simulink model "PubIfDecisionTOS_MDL"  (R2020b)
settings: configuration reference "DspaceConfig" (kept outside this file)
PostLoadFcn:
  | if any(exist('dsrtsu_mdlpostloadfcn', 'file') ~= 0), dsrtsu_mdlpostloadfcn('Execute', bdroot); end
InitFcn:
  | , if any(exist('dsmpb_private', 'file') ~= 0), dsmpb_private('dsmpb_mdlclblib', 'Init', bdroot); end,
undefined symbols (not defined in the file or in its folder): C_TOS_ACCEgoRAxletoFbumplength_m, C_TOS_ACCTargetFront_Flag, C_TOS_AEBJAPedObjDxThre_Val, C_TOS_AEBJAPedObjDyThre_Val, C_TOS_AEBJATargetSize_Val, C_TOS_AEBJAVehObjDxThre_Val, C_TOS_AEBJAVehObjDyThre_Val, C_TOS_AEBJuncPedTargetSize_Val, C_TOS_AEBLatObjDxThre_Val, C_TOS_AEBLatPedDyThre_Val, C_TOS_AEBLatTargetSize_Val, C_TOS_AEBLongTargetInEgoFront_Flag, C_TOS_axAbsGround_Parameter, C_TOS_CameraConfirmedFlag, C_TOS_CNsubjWidth, C_TOS_CurrentLaneCoreMinWidth_Val, C_TOS_CutInProb_Val_Zero, C_TOS_CutOutProb_Val_Zero, C_TOS_D2R_Val, C_TOS_DefaultValueObjectToCenterLine_dy, C_TOS_EgoCarWidth_Val, C_TOS_EgoDxRefPoint_m, C_TOS_EgoRAxletoFbumplength_m, C_TOS_HalfWidthVehicle_Con, C_TOS_HWA_CurrentLaneFlag, C_TOS_HWA_LeftLaneFlag, C_TOS_HWA_MovingDir_Vaild, C_TOS_HWA_MovState_Vaild, C_TOS_HWA_RightLaneFlag, C_TOS_LaneLineCourseErrorFront, C_TOS_LaneLineCourseErrorRear, C_TOS_MotorbikeDefaultWidth_m, C_TOS_NumberOfEffectiveTargets, C_TOS_Obj_Age_Val, C_TOS_Objdx_Constraint_Val, C_TOS_ObjectDefaultWidth_m, C_TOS_ObjInCurrentLane_Val, C_TOS_ObjInCurrentLaneValid, C_TOS_ObjInLeftLaneValid, C_TOS_ObjInRightLaneValid, C_TOS_ObjNotInCurrentLane_Val, C_TOS_ObjNotREElementType, C_TOS_ObjPredictDis_dy_ConstantVal_Zeros, C_TOS_ObjToCenterLine_ConstantVal_Zeros, C_TOS_OFMObjIDInvilad_Val, C_TOS_PIL_LatDisCons_Val_zero, C_TOS_PIL_ObjectCutInFlag_b, C_TOS_PIL_ObjectCutOutFlag_b, C_TOS_PIL_ObjLaneProb_al_Val, C_TOS_PP_ObjFusType_FC_Confirm_b, C_TOS_PP_ObjFusType_FC_FR_Confirm_b, C_TOS_PP_ObjFusType_FR_Confirm_b, C_TOS_RE_80BoolDefault_Val, C_TOS_RE_80Single181Default_Val, C_TOS_RE_80Single255Default_Val, C_TOS_RE_80Uint8Default_Val, C_TOS_RE_D2R, C_TOS_RE_D_180_Val, C_TOS_RE_InvalidObjectID_Val, C_TOS_RE_InvalidTargetChainDir_Val ... (+142)
libraries: simulink x1650, TOS_LIB x361, canfdmsglib x14
(part 15 of 69)

== system PubIfDecisionTOS_MDL/TOS_20201112/TOS_2012080320/PIL_1029/BoundaryCalculat/ObjectToCenterLine_dyc/SameLane/PIL_ObjectToCenterLine_dy_Filt ==
  note: fun: 目标到本车道中心线距离滤波
  TOS_OFMObjValid_Flag : Inport
  Object_ID : Inport  Port=2  OutDataTypeStr=uint8
  Object_Age : Inport  Port=3
  ObjectToCenterLine_dy : Inport  Port=4
  PIL_ObjectToCenterLine_dy : Subsystem
  Unit Delay : UnitDelay  InitialCondition=zeros(80,1)  SampleTime=-1  HasFrameUpgradeWarning=on
      settings: AttributesFormatString=initVal = zeros(80,1)
  Unit Delay1 : UnitDelay  InitialCondition=ones(80,1)*255  SampleTime=-1  HasFrameUpgradeWarning=on
      settings: AttributesFormatString=initVal = ones(80,1)*255
  PIL_ObjectToCenterLine_dy_Filt : Outport  OutDataTypeStr=single
  wires:
  TOS_OFMObjValid_Flag/1 -> PIL_ObjectToCenterLine_dy/4(TOS_OFMObjValid_Flag)
  Object_Age/1 -> PIL_ObjectToCenterLine_dy/6(Object_Age)
  ObjectToCenterLine_dy/1 -> PIL_ObjectToCenterLine_dy/3(ObjectToCenterLine_dy)
  PIL_ObjectToCenterLine_dy/2(ObjectToCenterLine_dy_Filt) -> PIL_ObjectToCenterLine_dy_Filt/1, Unit Delay1/1
  Unit Delay1/1 -> PIL_ObjectToCenterLine_dy/2(ObjectToCenterLine_dy_Filt_K1)
  Object_ID/1 -> PIL_ObjectToCenterLine_dy/5(Object_ID)
  PIL_ObjectToCenterLine_dy/1(Obj_ID) -> Unit Delay/1
  Unit Delay/1 -> PIL_ObjectToCenterLine_dy/1(ObjectID_Filt_K1)

== system PubIfDecisionTOS_MDL/TOS_20201112/TOS_2012080320/PIL_1029/BoundaryCalculat/ObjectToCenterLine_dyc/SameLane/SameCenterLine_dyc ==
  TOS_OFMObjValid_Flag : Inport  Partition=on  PartitionDimension=1  PartitionWidth=1  PartitionOffset=0
  Object_DY : Inport  Port=2  Partition=on  PartitionDimension=1  PartitionWidth=1  PartitionOffset=0
  Object_DX : Inport  Port=3  Partition=on  PartitionDimension=1  PartitionWidth=1  PartitionOffset=0
  line01_C0 : Inport  Port=4
  line01_C1 : Inport  Port=5
  line01_C2 : Inport  Port=6
  line01_C3 : Inport  Port=7
  line01_dDisStart : Inport  Port=8
  line01_dDisEnd : Inport  Port=9
  line02_C0 : Inport  Port=10
  line02_C1 : Inport  Port=11
  line02_C2 : Inport  Port=12
  line02_C3 : Inport  Port=13
  line02_dDisStart : Inport  Port=14
  line02_dDisEnd : Inport  Port=15
  line03_C0 : Inport  Port=16
  line03_C1 : Inport  Port=17
  line03_C2 : Inport  Port=18
  line03_C3 : Inport  Port=19
  line03_dDisStart : Inport  Port=20
  line03_dDisEnd : Inport  Port=21
  line04_C0 : Inport  Port=22
  line04_C1 : Inport  Port=23
  line04_C2 : Inport  Port=24
  line04_C3 : Inport  Port=25
  line04_dDisStart : Inport  Port=26
  line04_dDisEnd : Inport  Port=27
  line05_C0 : Inport  Port=28
  line05_C1 : Inport  Port=29
  line05_C2 : Inport  Port=30
  line05_C3 : Inport  Port=31
  line05_dDisStart : Inport  Port=32
  line05_dDisEnd : Inport  Port=33
  line06_C0 : Inport  Port=34
  line06_C1 : Inport  Port=35
  line06_C2 : Inport  Port=36
  line06_C3 : Inport  Port=37
  line06_dDisStart : Inport  Port=38
  line06_dDisEnd : Inport  Port=39
  Compare To Constant : simulink/Logic and Bit Operations/Compare To Constant  relop===  const=C_TOS_OFMObjIDInvilad_Val  OutDataTypeStr=boolean
      settings: AttributesFormatString=C_TOS_OFMObjIDInvilad_Val = 0
  For Each : ForEach  DisableCoverage=on
  If : If  IfExpression=u1 ~= 0
  Merge : Merge
  ObjToCenterLine_dyc_CurrentLane : Subsystem
  ObjToCenterLine_dyc_CurrentLaneDefault : Subsystem  TreatAsAtomicUnit=on
  SameCenterLine_dyc : Outport  ConcatenationDimension=1
  wires:
  ObjToCenterLine_dyc_CurrentLaneDefault/1(ObjectToCenterLine_dyc_CurrentLane) -> Merge/1
  Merge/1 -> SameCenterLine_dyc/1
  TOS_OFMObjValid_Flag/1 -> Compare To Constant/1
  If/2 -> ObjToCenterLine_dyc_CurrentLane/Action
  Compare To Constant/1 -> If/1
  If/1 -> ObjToCenterLine_dyc_CurrentLaneDefault/Action
  ObjToCenterLine_dyc_CurrentLane/1(ObjectToCenterLine_dyc_CurrentLane) -> Merge/2
  line06_dDisEnd/1 -> ObjToCenterLine_dyc_CurrentLane/38(line06_dDisEnd)
  line06_dDisStart/1 -> ObjToCenterLine_dyc_CurrentLane/37(line06_dDisStart)
  line06_C3/1 -> ObjToCenterLine_dyc_CurrentLane/36(line06_C3)
  line06_C2/1 -> ObjToCenterLine_dyc_CurrentLane/35(line06_C2)
  line06_C1/1 -> ObjToCenterLine_dyc_CurrentLane/34(line06_C1)
  line06_C0/1 -> ObjToCenterLine_dyc_CurrentLane/33(line06_C0)
  line05_dDisEnd/1 -> ObjToCenterLine_dyc_CurrentLane/32(line05_dDisEnd)
  line05_dDisStart/1 -> ObjToCenterLine_dyc_CurrentLane/31(line05_dDisStart)
  line05_C3/1 -> ObjToCenterLine_dyc_CurrentLane/30(line05_C3)
  line05_C2/1 -> ObjToCenterLine_dyc_CurrentLane/29(line05_C2)
  line05_C1/1 -> ObjToCenterLine_dyc_CurrentLane/28(line05_C1)
  line05_C0/1 -> ObjToCenterLine_dyc_CurrentLane/27(line05_C0)
  line04_dDisEnd/1 -> ObjToCenterLine_dyc_CurrentLane/26(line04_dDisEnd)
  line04_dDisStart/1 -> ObjToCenterLine_dyc_CurrentLane/25(line04_dDisStart)
  line04_C3/1 -> ObjToCenterLine_dyc_CurrentLane/24(line04_C3)
  line04_C2/1 -> ObjToCenterLine_dyc_CurrentLane/23(line04_C2)
  line04_C1/1 -> ObjToCenterLine_dyc_CurrentLane/22(line04_C1)
  line04_C0/1 -> ObjToCenterLine_dyc_CurrentLane/21(line04_C0)
  line03_dDisEnd/1 -> ObjToCenterLine_dyc_CurrentLane/20(line03_dDisEnd)
  line03_dDisStart/1 -> ObjToCenterLine_dyc_CurrentLane/19(line03_dDisStart)
  line03_C3/1 -> ObjToCenterLine_dyc_CurrentLane/18(line03_C3)
  line03_C2/1 -> ObjToCenterLine_dyc_CurrentLane/17(line03_C2)
  line03_C1/1 -> ObjToCenterLine_dyc_CurrentLane/16(line03_C1)
  line03_C0/1 -> ObjToCenterLine_dyc_CurrentLane/15(line03_C0)
  line02_dDisEnd/1 -> ObjToCenterLine_dyc_CurrentLane/14(line02_dDisEnd)
  line02_dDisStart/1 -> ObjToCenterLine_dyc_CurrentLane/13(line02_dDisStart)
  line02_C3/1 -> ObjToCenterLine_dyc_CurrentLane/12(line02_C3)
  line02_C2/1 -> ObjToCenterLine_dyc_CurrentLane/11(line02_C2)
  line02_C1/1 -> ObjToCenterLine_dyc_CurrentLane/10(line02_C1)
  line02_C0/1 -> ObjToCenterLine_dyc_CurrentLane/9(line02_C0)
  line01_dDisEnd/1 -> ObjToCenterLine_dyc_CurrentLane/8(line01_dDisEnd)
  line01_dDisStart/1 -> ObjToCenterLine_dyc_CurrentLane/7(line01_dDisStart)
  line01_C3/1 -> ObjToCenterLine_dyc_CurrentLane/6(line01_C3)
  line01_C2/1 -> ObjToCenterLine_dyc_CurrentLane/5(line01_C2)
  line01_C1/1 -> ObjToCenterLine_dyc_CurrentLane/4(line01_C1)
  line01_C0/1 -> ObjToCenterLine_dyc_CurrentLane/3(line01_C0)
  Object_DX/1 -> ObjToCenterLine_dyc_CurrentLane/2(Object_DX)
  Object_DY/1 -> ObjToCenterLine_dyc_CurrentLane/1(Object_DY)

== system PubIfDecisionTOS_MDL/TOS_20201112/TOS_2012080320/PIL_1029/ObjCutInOut_Prob/ObjectCutIn/CutInProb_Calculate/CutInProb_CalculateDefault ==
  Action Port : ActionPort  ActionPortLabel=if(u1 ~= 0)
  Constant1 : Constant  Value=0  OutDataTypeStr=single
  Constant2 : Constant  Value=0  OutDataTypeStr=single
  Constant3 : Constant  Value=255  OutDataTypeStr=single
  Constant4 : Constant  Value=0  OutDataTypeStr=boolean
  Constant5 : Constant  Value=255  OutDataTypeStr=single
  PIL_CutInPredictTime_ObserVale : Outport  OutDataTypeStr=single
  PIL_CutInPredictTime_dxConstraint_ObserVale : Outport  Port=2  OutDataTypeStr=single
  PIL_CutInPredictDis_dy_ObjWidthConstraint_ObserVale : Outport  Port=3
  PIL_ObjectCutinMindFlg_ObserVale : Outport  Port=4  OutDataTypeStr=boolean
  CutInProb_Calculate : Outport  Port=5
  wires:
  Constant2/1 -> PIL_CutInPredictTime_ObserVale/1
  Constant1/1 -> PIL_CutInPredictTime_dxConstraint_ObserVale/1
  Constant3/1 -> PIL_CutInPredictDis_dy_ObjWidthConstraint_ObserVale/1
  Constant4/1 -> PIL_ObjectCutinMindFlg_ObserVale/1
  Constant5/1 -> CutInProb_Calculate/1

== system PubIfDecisionTOS_MDL/TOS_20201112/TOS_2012080320/PIL_1029/ObjCutInOut_Prob/ObjectCutIn/CutInProb_Calculate/CutInProb_Calculate_ ==
  Object_Width : Inport  OutDataTypeStr=single
  Object_DX : Inport  Port=2  OutDataTypeStr=single
  Object_DY : Inport  Port=3  OutDataTypeStr=single
  Object_Age : Inport  Port=4  OutDataTypeStr=uint16
  Object_Type : Inport  Port=5
  PP_ObjectToCenterLine_dy : Inport  Port=6  OutDataTypeStr=single
  PP_ObjectToCenterLine_vyc : Inport  Port=7  OutDataTypeStr=single
  PIL_ObjectToCenterLine_dy_Filt : Inport  Port=8  OutDataTypeStr=single
  PP_CurrentLaneWidth : Inport  Port=9
  Action Port : ActionPort  ActionPortLabel=else
  Bus Creator : BusCreator  Inputs=9
  Bus Selector : BusSelector  OutputSignals=PIL_ObjectToCenterLine_dy_Filt,PP_ObjectToCenterLine_dy,Object_Type,Object_DX,PP_ObjectToCenterLine_vyc
  Bus Selector1 : BusSelector  OutputSignals=PP_ObjectToCenterLine_dy,Object_Width,Object_Type
  Bus Selector3 : BusSelector  OutputSignals=PP_ObjectToCenterLine_vyc,PP_ObjectToCenterLine_dy,PP_ObjectToCenterLine_dy,Object_Age,Object_Width
  CutInPredictDis_dy : Subsystem
  CutInProb : Subsystem
  CutInProb_ScopeConstraint : Subsystem
  CutInProb_ScopeConstraint1 : Subsystem  Commented=on
  PIL_CutInPredictTime_ObserVale : Outport  OutDataTypeStr=single
  PIL_CutInPredictTime_dxConstraint_ObserVale : Outport  Port=2  OutDataTypeStr=single
  PIL_CutInPredictDis_dy_ObjWidthConstraint_ObserVale : Outport  Port=3
  PIL_ObjectCutinMindFlg_ObserVale : Outport  Port=4  OutDataTypeStr=boolean
  CutInProb_Calculate : Outport  Port=5
  wires:
  Bus Selector1/3 -> CutInProb/4(ObjectType)  "<Object_Type>"
  CutInProb/2(CutInProb) -> CutInProb_ScopeConstraint/1(CutInProb)  "CutInProb"
  CutInProb/1(PIL_CutInPredictDis_dy_ObjWidthConstraint_ObserVale) -> PIL_CutInPredictDis_dy_ObjWidthConstraint_ObserVale/1
  PP_ObjectToCenterLine_vyc/1 -> Bus Creator/7  "PP_ObjectToCenterLine_vyc"
  Object_Age/1 -> Bus Creator/4  "Object_Age"
  CutInPredictDis_dy/3(CutInPredictDis_dy) -> CutInProb/1(CutInPredictDis_dy)  "CutInPredictDis_dy"
  Bus Selector1/2 -> CutInProb/3(Object_Width)  "<Object_Width>"
  CutInPredictDis_dy/2(PIL_CutInPredictTime_Constraint_ObserVale) -> PIL_CutInPredictTime_dxConstraint_ObserVale/1
  Bus Selector/1 -> CutInPredictDis_dy/1(ObjectToCenterLine_dy_Filt)  "<PIL_ObjectToCenterLine_dy_Filt>"
  Object_DY/1 -> Bus Creator/3  "Object_DY"
  Bus Selector/2 -> CutInPredictDis_dy/2(ObjectToCenterLine_dy)  "<PP_ObjectToCenterLine_dy>"
  Bus Selector1/1 -> CutInProb/2(ObjectToCenterLine_dy)  "<PP_ObjectToCenterLine_dy>"
  Bus Selector3/5 -> CutInProb_ScopeConstraint/6(Object_Width)  "<Object_Width>"
  [CutInProb_Calculate] -> Bus Selector3/1
  Bus Selector3/2 -> CutInProb_ScopeConstraint/3(ObjectToCenterLine_dy)  "<PP_ObjectToCenterLine_dy>"
  Bus Selector3/3 -> CutInProb_ScopeConstraint/4(PP_ObjectToCenterLine_dy)  "<PP_ObjectToCenterLine_dy>"
  Bus Selector3/4 -> CutInProb_ScopeConstraint/5(Object_Age)  "<Object_Age>"
  Bus Selector/4 -> CutInPredictDis_dy/4(Object_DX)  "<Object_DX>"
  Bus Selector/3 -> CutInPredictDis_dy/3(ObjectType)  "<Object_Type>"
  CutInProb_ScopeConstraint/1(PIL_ObjectCutinMindFlg_ObserVale) -> PIL_ObjectCutinMindFlg_ObserVale/1
  Object_Width/1 -> Bus Creator/1  "Object_Width"
  [CutInProb_Calculate] -> Bus Selector1/1
  CutInPredictDis_dy/1(PIL_CutInPredictTime_ObserVale) -> PIL_CutInPredictTime_ObserVale/1
  Object_Type/1 -> Bus Creator/5  "Object_Type"
  Bus Selector3/1 -> CutInProb_ScopeConstraint/2(PP_ObjectToCenterLine_vyc)  "<PP_ObjectToCenterLine_vyc>"
  Bus Creator/1 -> [CutInProb_Calculate], Bus Selector/1
  PP_ObjectToCenterLine_dy/1 -> Bus Creator/6  "PP_ObjectToCenterLine_dy"
  Object_DX/1 -> Bus Creator/2  "Object_DX"
  PIL_ObjectToCenterLine_dy_Filt/1 -> Bus Creator/8  "PIL_ObjectToCenterLine_dy_Filt"
  Bus Selector/5 -> CutInPredictDis_dy/5(PP_ObjectToCenterLine_vyc)  "<PP_ObjectToCenterLine_vyc>"
  CutInProb_ScopeConstraint/2(CutInProb_ScopeConstraint) -> CutInProb_Calculate/1
  PP_CurrentLaneWidth/1 -> Bus Creator/9  "PP_CurrentLaneWidth"

== system PubIfDecisionTOS_MDL/TOS_20201112/TOS_2012080320/PIL_1029/ObjCutInOut_Prob/ObjectCutIn/CutInProb_Pluse/CutInProb_Pluse ==
  note: 滤波处理
  CutInProb_Pluse_K1 : Inport  OutDataTypeStr=single
  CutInProb_ScopeConstraint : Inport  Port=2  OutDataTypeStr=single
  Object_Dx : Inport  Port=3  OutDataTypeStr=single
  Action Port : ActionPort  ActionPortLabel=if(u1 == 1)
  1-D Lookup Table : Lookup_n-D  NumberOfTableDimensions=1  BreakpointsForDimension1=[0,10,30,100]  Table=[0.25,0.25,0.4,0.4]  InternalRulePriority=Speed  RndMeth=Simplest  InputSameDT=on
  Abs : Abs  OutDataTypeStr=single
  Abs1 : Abs  OutDataTypeStr=single
  Add : Sum  Inputs=-+  AccumDataTypeStr=single
  Add1 : Sum  AccumDataTypeStr=single
  Add2 : Sum  Inputs=+-  AccumDataTypeStr=single
  Delay : Delay
  K_CutInPluseRate_Val : Constant  Value=P_TOS_CutInPluseUpperRate_Val
      settings: AttributesFormatString=P_TOS_CutInPluseUpperRate_Val = 0.7
  K_CutInPluseRate_Val1 : Constant  Value=P_TOS_CutInPluseDecreaseRate_Val
      settings: AttributesFormatString=P_TOS_CutInPluseDecreaseRate_Val = 0.2
  Logical Operator : Logic  Inputs=3  AllPortsSameDT=off  OutDataTypeStr=boolean
  Product : Product
  Product1 : Product
  Relational Operator2 : RelationalOperator  Operator=>  OutDataTypeStr=boolean  RndMeth=Nearest
  Switch : Switch  Criteria=u2 > Threshold  OutDataTypeStr=single
  Unit Delay : UnitDelay  SampleTime=-1  HasFrameUpgradeWarning=on
  PIL_CutInProb_Pluse : Outport  OutDataTypeStr=single
  PIL_ObjectCutInFlag : Outport  Port=2
  wires:
  Logical Operator/1 -> PIL_ObjectCutInFlag/1
  Delay/1 -> Logical Operator/3
  Unit Delay/1 -> Logical Operator/2
  Add/1 -> Abs1/1, Switch/2, Abs/1
  CutInProb_Pluse_K1/1 -> Add/1, Add2/1, Add1/1
  Switch/1 -> PIL_CutInProb_Pluse/1, Relational Operator2/1
  Add2/1 -> Switch/3
  K_CutInPluseRate_Val1/1 -> Product1/2
  Add1/1 -> Switch/1
  Abs/1 -> Product/2
  Object_Dx/1 -> 1-D Lookup Table/1
  Relational Operator2/1 -> Logical Operator/1, Delay/1, Unit Delay/1
  Product1/1 -> Add2/2
  CutInProb_ScopeConstraint/1 -> Add/2
  K_CutInPluseRate_Val/1 -> Product/1
  Abs1/1 -> Product1/1
  Product/1 -> Add1/2
  1-D Lookup Table/1 -> Relational Operator2/2  "P_TOS_ObjCutInProb_Val"

== system PubIfDecisionTOS_MDL/TOS_20201112/TOS_2012080320/PIL_1029/ObjCutInOut_Prob/ObjectCutIn/CutInProb_Pluse/CutInProb_PluseDefault ==
  Action Port : ActionPort  ActionPortLabel=else
  Constant1 : Constant  Value=0  OutDataTypeStr=boolean
  Constant2 : Constant  Value=0  OutDataTypeStr=single
  PIL_CutInProb_Pluse : Outport  OutDataTypeStr=single
  PIL_ObjectCutInFlag : Outport  Port=2
  wires:
  Constant2/1 -> PIL_CutInProb_Pluse/1
  Constant1/1 -> PIL_ObjectCutInFlag/1

== system PubIfDecisionTOS_MDL/TOS_20201112/TOS_2012080320/PIL_1029/ObjCutInOut_Prob/ObjectCutOut/CutOutProb_Calculate/CutOutProb_Calculate ==
  Object_Width : Inport
  Object_DX : Inport  Port=2
  Object_DY : Inport  Port=3
  Object_Age : Inport  Port=4
  Object_Type : Inport  Port=5
  PP_ObjectToCenterLine_dy : Inport  Port=6
  PP_ObjectToCenterLine_vyc : Inport  Port=7
  PIL_ObjectToCenterLine_dy_Filt : Inport  Port=8
  Object_VY : Inport  Port=9
  Action Port : ActionPort  ActionPortLabel=else
  Bus Creator : BusCreator  Inputs=9
  Bus Selector : BusSelector  OutputSignals=PIL_ObjectToCenterLine_dy_Filt,PP_ObjectToCenterLine_dy,Object_Type,Object_DX,PP_ObjectToCenterLine_vyc,Object_VY
  Bus Selector1 : BusSelector  OutputSignals=PIL_ObjectToCenterLine_dy_Filt,Object_Width,Object_Type
  Bus Selector3 : BusSelector  OutputSignals=PIL_ObjectToCenterLine_dy_Filt,PP_ObjectToCenterLine_vyc,PP_ObjectToCenterLine_dy,Object_Width,Object_Type
  CutOutPredictDis_dy : Subsystem
  CutOutProb : Subsystem
  CutOutProb_ScopeConstraint : Subsystem
  PIL_CutOutPredictTime_ObserVale : Outport  OutDataTypeStr=single
  PIL_CutOutPredictTime_dxConstraint_ObserVale : Outport  Port=2  OutDataTypeStr=single
  PIL_CutOutPredictDis_dy_ObjWidthConstraint_ObserVale : Outport  Port=3
  PIL_ObjectCutOutMindFlg_ObserVale : Outport  Port=4  OutDataTypeStr=boolean
  PIL_CutOutProb_ScopeConstraint : Outport  Port=5
  PIL_ObjectCutoutMindFlg1_ObserVale : Outport  Port=6  OutDataTypeStr=boolean
  PIL_ObjectCutoutMindFlg2_ObserVale : Outport  Port=7  OutDataTypeStr=boolean
  PIL_ObjectCutoutMindFlg3_ObserVale : Outport  Port=8  OutDataTypeStr=boolean
  wires:
  Bus Selector3/5 -> CutOutProb_ScopeConstraint/6(ObjectType)  "<Object_Type>"
  Bus Selector/6 -> CutOutPredictDis_dy/6(Object_VY)  "<Object_VY>"
  Object_VY/1 -> Bus Creator/9  "Object_VY"
  Bus Selector3/1 -> CutOutProb_ScopeConstraint/2(PIL_ObjectToCenterLine_dy_Filt)  "<PIL_ObjectToCenterLine_dy_Filt>"
  Bus Selector1/3 -> CutOutProb/4(ObjectType)  "<Object_Type>"
  CutOutPredictDis_dy/2(PIL_CutOutPredictTime_dxConstraint_ObserVale) -> PIL_CutOutPredictTime_dxConstraint_ObserVale/1
  PP_ObjectToCenterLine_vyc/1 -> Bus Creator/7  "PP_ObjectToCenterLine_vyc"
  PP_ObjectToCenterLine_dy/1 -> Bus Creator/6  "PP_ObjectToCenterLine_dy"
  Bus Selector3/3 -> CutOutProb_ScopeConstraint/4(PP_ObjectToCenterLine_dy)  "<PP_ObjectToCenterLine_dy>"
  Bus Selector1/1 -> CutOutProb/2(PIL_ObjectToCenterLine_dy_Filt)  "<PIL_ObjectToCenterLine_dy_Filt>"
  CutOutPredictDis_dy/3(CutOutPredictDis_dy) -> CutOutProb/1(CutOutPredictDis_dy)
  Bus Selector/2 -> CutOutPredictDis_dy/2(ObjectToCenterLine_dy)  "<PP_ObjectToCenterLine_dy>"
  Object_Age/1 -> Bus Creator/4  "Object_Age"
  PIL_ObjectToCenterLine_dy_Filt/1 -> Bus Creator/8  "PIL_ObjectToCenterLine_dy_Filt"
  Bus Selector/5 -> CutOutPredictDis_dy/5(PP_ObjectToCenterLine_vyc)  "<PP_ObjectToCenterLine_vyc>"
  Bus Selector/3 -> CutOutPredictDis_dy/3(ObjectType)  "<Object_Type>"
  Bus Selector/4 -> CutOutPredictDis_dy/4(Object_DX)  "<Object_DX>"
  [CutOutProb_Calculate] -> Bus Selector3/1
  CutOutPredictDis_dy/1(PIL_CutOutPredictTime_ObserVale) -> PIL_CutOutPredictTime_ObserVale/1
  Bus Selector1/2 -> CutOutProb/3(Object_Width)  "<Object_Width>"
  Object_Type/1 -> Bus Creator/5  "Object_Type"
  Object_Width/1 -> Bus Creator/1  "Object_Width"
  Bus Selector3/2 -> CutOutProb_ScopeConstraint/3(PP_ObjectToCenterLine_vyc)  "<PP_ObjectToCenterLine_vyc>"
  Bus Selector/1 -> CutOutPredictDis_dy/1(ObjectToCenterLine_dy_Filt)  "<PIL_ObjectToCenterLine_dy_Filt>"
  Bus Creator/1 -> [CutOutProb_Calculate], Bus Selector/1
  Object_DX/1 -> Bus Creator/2  "Object_DX"
  Bus Selector3/4 -> CutOutProb_ScopeConstraint/5(Object_Width)  "<Object_Width>"
  CutOutProb/2(CutOutProb) -> CutOutProb_ScopeConstraint/1(CutOutProb)  "CutOutProb"
  Object_DY/1 -> Bus Creator/3  "Object_DY"
  CutOutProb_ScopeConstraint/2(CutOutProb_ScopeConstraint) -> PIL_CutOutProb_ScopeConstraint/1
  [CutOutProb_Calculate] -> Bus Selector1/1
  CutOutProb_ScopeConstraint/1(PIL_ObjectCutOutMindFlg_ObserVale) -> PIL_ObjectCutOutMindFlg_ObserVale/1
  CutOutProb/1(PIL_CutOutPredictDis_dy_ObjWidthConstraint_ObserVale) -> PIL_CutOutPredictDis_dy_ObjWidthConstraint_ObserVale/1
  CutOutProb_ScopeConstraint/3(PIL_ObjectCutoutMindFlg1_ObserVale) -> PIL_ObjectCutoutMindFlg1_ObserVale/1
  CutOutProb_ScopeConstraint/4(PIL_ObjectCutoutMindFlg2_ObserVale) -> PIL_ObjectCutoutMindFlg2_ObserVale/1
  CutOutProb_ScopeConstraint/5(PIL_ObjectCutoutMindFlg3_ObserVale) -> PIL_ObjectCutoutMindFlg3_ObserVale/1

== system PubIfDecisionTOS_MDL/TOS_20201112/TOS_2012080320/PIL_1029/ObjCutInOut_Prob/ObjectCutOut/CutOutProb_Calculate/CutOutProb_CalculateDefault ==
  Action Port : ActionPort  ActionPortLabel=if(u1 ~= 0)
  Constant1 : Constant  Value=0  OutDataTypeStr=single
  Constant2 : Constant  Value=0  OutDataTypeStr=single
  Constant3 : Constant  Value=255  OutDataTypeStr=single
  Constant{4,6..8} (4 alike) : Constant  Value=0  OutDataTypeStr=boolean
  Constant5 : Constant  Value=255  OutDataTypeStr=single
  PIL_CutOutPredictTime_ObserVale : Outport  OutDataTypeStr=single
  PIL_CutOutPredictTime_Constraint_ObserVale : Outport  Port=2  OutDataTypeStr=single
  PIL_CutOutPredictDis_dy_ObjWidthConstraint_ObserVale : Outport  Port=3
  PIL_ObjectCutOutMindFlg_ObserVale : Outport  Port=4  OutDataTypeStr=boolean
  PIL_CutOutProb_ScopeConstraint : Outport  Port=5
  PIL_ObjectCutoutMindFlg1_ObserVale : Outport  Port=6  OutDataTypeStr=boolean
  PIL_ObjectCutoutMindFlg2_ObserVale : Outport  Port=7  OutDataTypeStr=boolean
  PIL_ObjectCutoutMindFlg3_ObserVale : Outport  Port=8  OutDataTypeStr=boolean
  wires:
  Constant5/1 -> PIL_CutOutProb_ScopeConstraint/1
  Constant4/1 -> PIL_ObjectCutOutMindFlg_ObserVale/1
  Constant3/1 -> PIL_CutOutPredictDis_dy_ObjWidthConstraint_ObserVale/1
  Constant1/1 -> PIL_CutOutPredictTime_Constraint_ObserVale/1
  Constant2/1 -> PIL_CutOutPredictTime_ObserVale/1
  Constant6/1 -> PIL_ObjectCutoutMindFlg1_ObserVale/1
  Constant7/1 -> PIL_ObjectCutoutMindFlg2_ObserVale/1
  Constant8/1 -> PIL_ObjectCutoutMindFlg3_ObserVale/1

== system PubIfDecisionTOS_MDL/TOS_20201112/TOS_2012080320/PIL_1029/ObjCutInOut_Prob/ObjectCutOut/CutOutProb_Pluse/CutInProb_PluseDefault ==
  Action Port : ActionPort  ActionPortLabel=else
  Constant1 : Constant  Value=0  OutDataTypeStr=boolean
  Constant2 : Constant  Value=0  OutDataTypeStr=single
  PIL_CutOutProb_Pluse : Outport  OutDataTypeStr=single
  PIL_ObjectCutOutFlag : Outport  Port=2
  wires:
  Constant2/1 -> PIL_CutOutProb_Pluse/1
  Constant1/1 -> PIL_ObjectCutOutFlag/1

== system PubIfDecisionTOS_MDL/TOS_20201112/TOS_2012080320/PIL_1029/ObjCutInOut_Prob/ObjectCutOut/CutOutProb_Pluse/Subsystem ==
  note: 滤波处理
  CutOutProb_Pluse_K1 : Inport  OutDataTypeStr=single
  CutOutProb_ScopeConstraint : Inport  Port=2  OutDataTypeStr=single
  Action Port : ActionPort  ActionPortLabel=if(u1 == 1)
  Abs : Abs  OutDataTypeStr=single
  Abs1 : Abs  OutDataTypeStr=single
  Add : Sum  Inputs=-+  AccumDataTypeStr=single
  Add1 : Sum  AccumDataTypeStr=single
  Add2 : Sum  Inputs=+-  AccumDataTypeStr=single
  Constant1 : Constant  Value=P_TOS_ObjCutOutProb_Val
      settings: AttributesFormatString=P_TOS_ObjCutOutProb_Val = 0.7
  Delay : Delay
  K_CutInPluseRate_Val : Constant  Value=P_TOS_CutOutPluseUpperRate_Val
      settings: AttributesFormatString=P_TOS_CutOutPluseUpperRate_Val = 0.2
  K_CutInPluseRate_Val1 : Constant  Value=P_TOS_CutOutPluseDecreaseRate_Val
      settings: AttributesFormatString=P_TOS_CutOutPluseDecreaseRate_Val = 0.2
  Logical Operator : Logic  Inputs=3  AllPortsSameDT=off  OutDataTypeStr=boolean
  Product : Product
  Product1 : Product
  Relational Operator2 : RelationalOperator  Operator=>  OutDataTypeStr=boolean  RndMeth=Nearest
  Switch : Switch  Criteria=u2 > Threshold  OutDataTypeStr=single
  Unit Delay : UnitDelay  SampleTime=-1  HasFrameUpgradeWarning=on
  PIL_CutOutProb_Pluse : Outport  OutDataTypeStr=single
  PIL_ObjectCutOutFlag : Outport  Port=2
  wires:
  Logical Operator/1 -> PIL_ObjectCutOutFlag/1
  Relational Operator2/1 -> Logical Operator/1, Delay/1, Unit Delay/1
  Delay/1 -> Logical Operator/3
  Unit Delay/1 -> Logical Operator/2
  CutOutProb_Pluse_K1/1 -> Add1/1, Add2/1, Add/1
  Add/1 -> Abs1/1, Switch/2, Abs/1
  K_CutInPluseRate_Val/1 -> Product/1
  Constant1/1 -> Relational Operator2/2
  Add2/1 -> Switch/3
  CutOutProb_ScopeConstraint/1 -> Add/2
  Switch/1 -> PIL_CutOutProb_Pluse/1, Relational Operator2/1
  Add1/1 -> Switch/1
  Product1/1 -> Add2/2
  Abs1/1 -> Product1/1
  K_CutInPluseRate_Val1/1 -> Product1/2
  Abs/1 -> Product/2
  Product/1 -> Add1/2

== system PubIfDecisionTOS_MDL/TOS_20201112/TOS_2012080320/PIL_1029/ProbCalculat/ProbCalculat/ObjectProbCalculation/ProbCalculation ==
  Object_Width : Inport
  Object_Type : Inport  Port=2
  PIL_SameCenterLine_dyc : Inport  Port=3
  PIL_LeftCenterLine_dyc : Inport  Port=4
  PIL_RightCenterLine_dyc : Inport  Port=5
  SameLane_CoreArea_Boundary : Inport  Port=6
  SameLane_EdgeLeft_Boundary : Inport  Port=7
  SameLane_EdgeRight_Boundary : Inport  Port=8
  LeftLane_CoreArea_Boundary : Inport  Port=9
  LeftLane_EdgeLeft_Boundary : Inport  Port=10
  LeftLane_EdgeRight_Boundary : Inport  Port=11
  RightLane_CoreArea_Boundary : Inport  Port=12
  RightLane_EdgeLeft_Boundary : Inport  Port=13
  RightLane_EdgeRight_Boundary : Inport  Port=14
  Action Port : ActionPort  ActionPortLabel=else
  Add : Sum  Inputs=+++  OutDataTypeStr=single
  Bus Creator : BusCreator  Inputs=14
  Bus Selector : BusSelector  OutputSignals=PIL_SameCenterLine_dyc,SameLane_CoreArea_Boundary,SameLane_EdgeLeft_Boundary
  Bus Selector1 : BusSelector  OutputSignals=PIL_SameCenterLine_dyc
  Bus Selector2 : BusSelector  OutputSignals=PIL_SameCenterLine_dyc,SameLane_CoreArea_Boundary,SameLane_EdgeRight_Boundary
  Bus Selector3 : BusSelector  OutputSignals=PIL_LeftCenterLine_dyc,LeftLane_CoreArea_Boundary,LeftLane_EdgeLeft_Boundary
  Bus Selector4 : BusSelector  OutputSignals=PIL_LeftCenterLine_dyc
  Bus Selector5 : BusSelector  OutputSignals=PIL_LeftCenterLine_dyc,LeftLane_CoreArea_Boundary,LeftLane_EdgeRight_Boundary
  Bus Selector6 : BusSelector  OutputSignals=PIL_RightCenterLine_dyc
  Bus Selector7 : BusSelector  OutputSignals=PIL_RightCenterLine_dyc,RightLane_CoreArea_Boundary,RightLane_EdgeLeft_Boundary
  Bus Selector8 : BusSelector  OutputSignals=PIL_RightCenterLine_dyc,RightLane_CoreArea_Boundary,RightLane_EdgeRight_Boundary
  Compare To Constant : simulink/Logic and Bit Operations/Compare To Constant  relop=>  const=C_TOS_ObjToCenterLine_ConstantVal_Zeros  OutDataTypeStr=boolean
      settings: AttributesFormatString=C_TOS_ObjToCenterLine_ConstantVal_Zeros = 0
  Compare To Constant1 : simulink/Logic and Bit Operations/Compare To Constant  relop=>  const=C_TOS_ObjToCenterLine_ConstantVal_Zeros  OutDataTypeStr=boolean
      settings: AttributesFormatString=C_TOS_ObjToCenterLine_ConstantVal_Zeros = 0
  Compare To Constant2 : simulink/Logic and Bit Operations/Compare To Constant  relop=>  const=C_TOS_ObjToCenterLine_ConstantVal_Zeros  OutDataTypeStr=boolean
      settings: AttributesFormatString=C_TOS_ObjToCenterLine_ConstantVal_Zeros = 0
  LeftLane_LeftPro : Subsystem
  LeftLane_RightPro : Subsystem
  RightLane_LeftPro : Subsystem
  RightLane_RightPro : Subsystem
  SameLane_LeftPro : Subsystem
  SameLane_RightPro : Subsystem
  Switch1 : Switch  Criteria=u2 ~= 0  OutDataTypeStr=single
  Switch2 : Switch  Criteria=u2 ~= 0  OutDataTypeStr=single
  Switch3 : Switch  Criteria=u2 ~= 0  OutDataTypeStr=single
  "PIL_ObjLaneProb _all " : Outport
  PIL_EgoLaneProb : Outport  Port=2  InitialOutput=0
  PIL_LeftLaneProb : Outport  Port=3
  PIL_RightLaneProb : Outport  Port=4
  wires:
  Bus Selector8/3 -> RightLane_RightPro/3(RightLane_EdgeRight_Boundary)  "<RightLane_EdgeRight_Boundary>"
  Bus Selector8/2 -> RightLane_RightPro/2(RightLane_CoreArea_Boundary)  "<RightLane_CoreArea_Boundary>"
  Bus Selector8/1 -> RightLane_RightPro/1(PIL_RightCenterLine_dyc)  "<PIL_RightCenterLine_dyc>"
  RightLane_RightPro/1(RightLane_RightPro) -> Switch3/3
  RightLane_LeftPro/1(RightLane_LeftPro) -> Switch3/1
  Bus Creator/1 -> Bus Selector/1, Bus Selector1/1, Bus Selector2/1, Bus Selector4/1, Bus Selector5/1, Bus Selector7/1, Bus Selector6/1, Bus Selector8/1, Bus Selector3/1
  Bus Selector7/1 -> RightLane_LeftPro/1(PIL_RightCenterLine_dyc)  "<PIL_RightCenterLine_dyc>"
  Bus Selector7/3 -> RightLane_LeftPro/3(RightLane_EdgeLeft_Boundary)  "<RightLane_EdgeLeft_Boundary>"
  Bus Selector7/2 -> RightLane_LeftPro/2(RightLane_CoreArea_Boundary)  "<RightLane_CoreArea_Boundary>"
  Switch3/1 -> PIL_RightLaneProb/1, Add/1  "PIL_RightLaneProb"
  Compare To Constant2/1 -> Switch3/2
  Bus Selector6/1 -> Compare To Constant2/1  "<PIL_RightCenterLine_dyc>"
  Switch1/1 -> Add/2, PIL_LeftLaneProb/1  "PIL_LeftLaneProb"
  Bus Selector5/3 -> LeftLane_RightPro/3(LeftLane_EdgeRight_Boundary)  "<LeftLane_EdgeRight_Boundary>"
  Bus Selector5/2 -> LeftLane_RightPro/2(LeftLane_CoreArea_Boundary)  "<LeftLane_CoreArea_Boundary>"
  Bus Selector5/1 -> LeftLane_RightPro/1(PIL_LeftCenterLine_dyc)  "<PIL_LeftCenterLine_dyc>"
  LeftLane_RightPro/1(LeftLane_RightPro) -> Switch1/3
  LeftLane_LeftPro/1(LeftLane_LeftPro) -> Switch1/1
  Bus Selector3/2 -> LeftLane_LeftPro/2(LeftLane_CoreArea_Boundary)  "<LeftLane_CoreArea_Boundary>"
  Bus Selector3/3 -> LeftLane_LeftPro/3(LeftLane_EdgeLeft_Boundary)  "<LeftLane_EdgeLeft_Boundary>"
  Bus Selector3/1 -> LeftLane_LeftPro/1(PIL_LeftCenterLine_dyc)  "<PIL_LeftCenterLine_dyc>"
  Compare To Constant1/1 -> Switch1/2
  Bus Selector4/1 -> Compare To Constant1/1  "<PIL_LeftCenterLine_dyc>"
  RightLane_EdgeRight_Boundary/1 -> Bus Creator/14  "RightLane_EdgeRight_Boundary"
  RightLane_EdgeLeft_Boundary/1 -> Bus Creator/13  "RightLane_EdgeLeft_Boundary"
  RightLane_CoreArea_Boundary/1 -> Bus Creator/12  "RightLane_CoreArea_Boundary"
  LeftLane_EdgeRight_Boundary/1 -> Bus Creator/11  "LeftLane_EdgeRight_Boundary"
  LeftLane_EdgeLeft_Boundary/1 -> Bus Creator/10  "LeftLane_EdgeLeft_Boundary"
  LeftLane_CoreArea_Boundary/1 -> Bus Creator/9  "LeftLane_CoreArea_Boundary"
  PIL_RightCenterLine_dyc/1 -> Bus Creator/5  "PIL_RightCenterLine_dyc"
  PIL_LeftCenterLine_dyc/1 -> Bus Creator/4  "PIL_LeftCenterLine_dyc"
  Bus Selector2/3 -> SameLane_RightPro/3(SameLane_EdgeRight_Boundary)  "<SameLane_EdgeRight_Boundary>"
  Bus Selector2/2 -> SameLane_RightPro/2(SameLane_CoreArea_Boundary)  "<SameLane_CoreArea_Boundary>"
  Bus Selector2/1 -> SameLane_RightPro/1(PIL_SameCenterLine_dyc)  "<PIL_SameCenterLine_dyc>"
  SameLane_RightPro/1(SameLane_RightPro) -> Switch2/3
  Bus Selector/3 -> SameLane_LeftPro/3(SameLane_EdgeLeft_Boundary)  "<SameLane_EdgeLeft_Boundary>"
  Bus Selector/2 -> SameLane_LeftPro/2(SameLane_CoreArea_Boundary)  "<SameLane_CoreArea_Boundary>"
  Bus Selector/1 -> SameLane_LeftPro/1(PIL_SameCenterLine_dyc)  "<PIL_SameCenterLine_dyc>"
  Bus Selector1/1 -> Compare To Constant/1  "<PIL_SameCenterLine_dyc>"
  SameLane_EdgeLeft_Boundary/1 -> Bus Creator/7  "SameLane_EdgeLeft_Boundary"
  SameLane_CoreArea_Boundary/1 -> Bus Creator/6  "SameLane_CoreArea_Boundary"
  PIL_SameCenterLine_dyc/1 -> Bus Creator/3  "PIL_SameCenterLine_dyc"
  Object_Type/1 -> Bus Creator/2  "Object_Type"
  SameLane_EdgeRight_Boundary/1 -> Bus Creator/8  "SameLane_EdgeRight_Boundary"
  Object_Width/1 -> Bus Creator/1  "Object_Width"
  Compare To Constant/1 -> Switch2/2
  Switch2/1 -> Add/3, PIL_EgoLaneProb/1  "PIL_EgoLaneProb"
  SameLane_LeftPro/1(SameLane_LeftPro) -> Switch2/1
  Add/1 -> "PIL_ObjLaneProb _all "/1

== system PubIfDecisionTOS_MDL/TOS_20201112/TOS_2012080320/PIL_1029/ProbCalculat/ProbCalculat/ObjectProbCalculation/ProbCalculationDefault ==
  Action Port : ActionPort  ActionPortLabel=if(u1 ~= 0)
  Constant{1..4} (4 alike) : Constant  Value=0  OutDataTypeStr=single
  "PIL_ObjLaneProb _all " : Outport  OutDataTypeStr=single
  PIL_EgoLaneProb : Outport  Port=2  OutDataTypeStr=single
  PIL_LeftLaneProb : Outport  Port=3
  PIL_RightLaneProb : Outport  Port=4
  wires:
  Constant3/1 -> PIL_RightLaneProb/1
  Constant1/1 -> PIL_LeftLaneProb/1
  Constant2/1 -> PIL_EgoLaneProb/1
  Constant4/1 -> "PIL_ObjLaneProb _all "/1

== system PubIfDecisionTOS_MDL/TOS_20201112/TOS_2012080320/PIL_1029/ProbCalculat/ProbCalculat/Subsystem/EgoVehiclePro ==
  LL_C0 : Inport  Partition=on  PartitionDimension=1  PartitionWidth=1  PartitionOffset=0
  LR_C0 : Inport  Port=2  Partition=on  PartitionDimension=1  PartitionWidth=1  PartitionOffset=0
  RL_C0 : Inport  Port=3  Partition=on  PartitionDimension=1  PartitionWidth=1  PartitionOffset=0
  RR_C0 : Inport  Port=4  Partition=on  PartitionDimension=1  PartitionWidth=1  PartitionOffset=0
  HalfEgoWidth : Inport  Port=5
  Bus Creator1 : BusCreator  Inputs=5
  Bus Selector : BusSelector  OutputSignals=HalfEgoWidth,LL_C0,LR_C0
  Bus Selector1 : BusSelector  OutputSignals=HalfEgoWidth,LR_C0,RL_C0
  Bus Selector2 : BusSelector  OutputSignals=HalfEgoWidth,RL_C0,RR_C0
  EgoLaneProb : Subsystem
  For Each : ForEach  DisableCoverage=on
  LeftLaneProb : Subsystem
  RightLaneProb : Subsystem
  EgoVehicle_LeftLaneProb : Outport  ConcatenationDimension=1
  EgoVehicle_EgoLaneProb : Outport  Port=2  ConcatenationDimension=1
  EgoVehicle_RightLaneProb : Outport  Port=3  ConcatenationDimension=1
  wires:
  LeftLaneProb/1(" LeftLaneProb") -> EgoVehicle_LeftLaneProb/1  "EgoVehicle_LeftLaneProb"
  RightLaneProb/1(" RightLaneProb") -> EgoVehicle_RightLaneProb/1  "EgoVehicle_RightLaneProb"
  EgoLaneProb/1(" EgoLaneProb") -> EgoVehicle_EgoLaneProb/1  "EgoVehicle_EgoLaneProb"
  HalfEgoWidth/1 -> Bus Creator1/1  "HalfEgoWidth"
  LL_C0/1 -> Bus Creator1/2  "LL_C0"
  LR_C0/1 -> Bus Creator1/3  "LR_C0"
  RL_C0/1 -> Bus Creator1/4  "RL_C0"
  RR_C0/1 -> Bus Creator1/5  "RR_C0"
  Bus Creator1/1 -> Bus Selector1/1, Bus Selector2/1, Bus Selector/1
  Bus Selector/1 -> LeftLaneProb/1(HalfEgoWidth)  "<HalfEgoWidth>"
  Bus Selector/2 -> LeftLaneProb/2(t_dleft_LeftLane)  "<LL_C0>"
  Bus Selector/3 -> LeftLaneProb/3(t_dright_LeftLane)  "<LR_C0>"
  Bus Selector1/1 -> EgoLaneProb/1(HalfEgoWidth)  "<HalfEgoWidth>"
  Bus Selector1/2 -> EgoLaneProb/2(t_dleft_EgoLane)  "<LR_C0>"
  Bus Selector1/3 -> EgoLaneProb/3(t_dright_EgoLane)  "<RL_C0>"
  Bus Selector2/1 -> RightLaneProb/1(HalfEgoWidth)  "<HalfEgoWidth>"
  Bus Selector2/2 -> RightLaneProb/2(t_dleft_RightLane)  "<RL_C0>"
  Bus Selector2/3 -> RightLaneProb/3(t_dright_RightLane)  "<RR_C0>"

== system PubIfDecisionTOS_MDL/TOS_20201112/TOS_2012080320/PIL_1029/ProbCalculat/ProbCalculat/Subsystem/PIL_EgoVehiclePro ==
  PIL_EgoVehiclePro : Inport
  Bus Creator : BusCreator  Inputs=3  OutDataTypeStr=Bus: EgoVehicleProCalcu_BUS  NonVirtualBus=on
      settings: InheritFromInputs=off
  Bus Selector4 : BusSelector  OutputSignals=EgoVehicle_LeftLaneProb,EgoVehicle_EgoLaneProb,EgoVehicle_RightLaneProb
  EgoVehicle_EgoLaneProb : Subsystem
  EgoVehicle_LeftLaneProb : Subsystem
  EgoVehicle_RightLaneProb : Subsystem
  PIL_EgoVehicleProFilt : Outport
  wires:
  Bus Creator/1 -> PIL_EgoVehicleProFilt/1
  EgoVehicle_RightLaneProb/1(EgoVehicle_RightLaneProb_Filt) -> Bus Creator/3  "EgoCar_RightLaneProb"
  EgoVehicle_LeftLaneProb/1(EgoVehicle_LeftLaneProb_Filt) -> Bus Creator/1  "EgoCar_LeftLaneProb"
  EgoVehicle_EgoLaneProb/1(EgoCar_CurrentLaneProb_Filt) -> Bus Creator/2  "EgoCar_CurrentLaneProb"
  Bus Selector4/1 -> EgoVehicle_LeftLaneProb/1(EgoVehicle_LeftLaneProb)  "<EgoVehicle_LeftLaneProb>"
  Bus Selector4/2 -> EgoVehicle_EgoLaneProb/1(EgoCar_CurrentLaneProb)  "<EgoVehicle_EgoLaneProb>"
  Bus Selector4/3 -> EgoVehicle_RightLaneProb/1(EgoVehicle_RightLaneProb)  "<EgoVehicle_RightLaneProb>"
  PIL_EgoVehiclePro/1 -> Bus Selector4/1

== system PubIfDecisionTOS_MDL/TOS_20201112/TOS_2012080320/PP1128/AAT-AdditionalAttributes/PP_CenterLine_Calculat/EgoLane_CenterLine/EgoLaneCenterLine01 ==
  EgoLaneLine : Inport
  Add{,1..3} (4 alike) : Sum
  Bus Creator : BusCreator  Inputs=6
  Bus Selector : BusSelector  OutputSignals=TOS_LM_LR_Bus.LM_LR_Line01.pC0,TOS_LM_RL_Bus.LM_RL_Line01.pC0
  Bus Selector1 : BusSelector  OutputSignals=TOS_LM_LR_Bus.LM_LR_Line01.pC3,TOS_LM_RL_Bus.LM_RL_Line01.pC3
  Bus Selector3 : BusSelector  OutputSignals=TOS_LM_LR_Bus.LM_LR_Line01.pC1,TOS_LM_RL_Bus.LM_RL_Line01.pC1
  Bus Selector4 : BusSelector  OutputSignals=TOS_LM_LR_Bus.LM_LR_Line01.dDisStart,TOS_LM_LR_Bus.LM_LR_Line01.dDisEnd
  Bus Selector5 : BusSelector  OutputSignals=TOS_LM_LR_Bus.LM_LR_Line01.pC2,TOS_LM_RL_Bus.LM_RL_Line01.pC2
  Data{,1..3} (4 alike) : TOS_LIB/Data  SystemSampleTime=-1  VariantActivationTime=update diagram  Latency=0  AutoFrameSizeCalculation=off
  Gain{1..4} (4 alike) : Gain  Gain=0.5  ParamDataTypeStr=single  OutDataTypeStr=single
  Signal Copy1 : SignalConversion  OverrideOpt=off
  Signal Copy2 : SignalConversion  OverrideOpt=off
  EgoLaneCenterLine01 : Outport
  wires:
  EgoLaneLine/1 -> Bus Selector4/1, Bus Selector/1, Bus Selector3/1, Bus Selector5/1, Bus Selector1/1
  Bus Selector/1 -> Add/1  "<pC0>"
  Bus Selector/2 -> Add/2  "<pC0>"
  Add/1 -> Gain4/1
  Data3/1 -> Bus Creator/4  "PC0"
  Add1/1 -> Gain1/1
  Bus Selector1/2 -> Add1/2  "<pC3>"
  Bus Selector1/1 -> Add1/1  "<pC3>"
  Bus Selector5/1 -> Add2/1  "<pC2>"
  Bus Selector5/2 -> Add2/2  "<pC2>"
  Add2/1 -> Gain2/1
  Add3/1 -> Gain3/1
  Bus Selector3/2 -> Add3/2  "<pC1>"
  Bus Selector3/1 -> Add3/1  "<pC1>"
  Data/1 -> Bus Creator/1  "PC3"
  Bus Creator/1 -> EgoLaneCenterLine01/1  "CenterLine01"
  Data2/1 -> Bus Creator/3  "PC1"
  Data1/1 -> Bus Creator/2  "PC2"
  Bus Selector4/1 -> Signal Copy2/1  "<dDisStart>"
  Bus Selector4/2 -> Signal Copy1/1  "<dDisEnd>"
  Signal Copy2/1 -> Data3/2, Data1/2, Data/2, Data2/2, Bus Creator/5  "dDisStart"
  Signal Copy1/1 -> Data3/3, Data2/3, Data1/3, Data/3, Bus Creator/6  "dDisEnd"
  Gain2/1 -> Data1/1  "PC2"
  Gain1/1 -> Data/1  "PC3"
  Gain4/1 -> Data3/1  "PC0"
  Gain3/1 -> Data2/1  "PC1"

== system PubIfDecisionTOS_MDL/TOS_20201112/TOS_2012080320/PP1128/AAT-AdditionalAttributes/PP_CenterLine_Calculat/EgoLane_CenterLine/EgoLaneCenterLine02 ==
  EgoLaneLine : Inport
  Add{,1..3} (4 alike) : Sum
  Bus Creator : BusCreator  Inputs=6
  Bus Selector : BusSelector  OutputSignals=TOS_LM_LR_Bus.LM_LR_Line02.pC0,TOS_LM_RL_Bus.LM_RL_Line02.pC0
  Bus Selector1 : BusSelector  OutputSignals=TOS_LM_LR_Bus.LM_LR_Line02.pC3,TOS_LM_RL_Bus.LM_RL_Line02.pC3
  Bus Selector2 : BusSelector  OutputSignals=TOS_LM_LR_Bus.LM_LR_Line02.pC2,TOS_LM_RL_Bus.LM_RL_Line02.pC2
  Bus Selector3 : BusSelector  OutputSignals=TOS_LM_LR_Bus.LM_LR_Line02.pC1,TOS_LM_RL_Bus.LM_RL_Line02.pC1
  Bus Selector4 : BusSelector  OutputSignals=TOS_LM_LR_Bus.LM_LR_Line02.dDisStart,TOS_LM_LR_Bus.LM_LR_Line02.dDisEnd
  Data{,1..3} (4 alike) : TOS_LIB/Data  SystemSampleTime=-1  VariantActivationTime=update diagram  Latency=0  AutoFrameSizeCalculation=off
  Gain{1..4} (4 alike) : Gain  Gain=0.5  ParamDataTypeStr=single  OutDataTypeStr=single
  Signal Copy1 : SignalConversion  OverrideOpt=off
  Signal Copy2 : SignalConversion  OverrideOpt=off
  EgoLaneCenterLine02 : Outport
  wires:
  Bus Selector/1 -> Add/1  "<pC0>"
  Add/1 -> Gain4/1
  Bus Selector/2 -> Add/2  "<pC0>"
  Bus Selector1/2 -> Add1/2  "<pC3>"
  Bus Selector3/2 -> Add3/2  "<pC1>"
  Add1/1 -> Gain1/1
  Bus Selector1/1 -> Add1/1  "<pC3>"
  Bus Selector2/2 -> Add2/2  "<pC2>"
  Add3/1 -> Gain3/1
  Bus Selector2/1 -> Add2/1  "<pC2>"
  EgoLaneLine/1 -> Bus Selector1/1, Bus Selector2/1, Bus Selector3/1, Bus Selector4/1, Bus Selector/1
  Bus Selector3/1 -> Add3/1  "<pC1>"
  Add2/1 -> Gain2/1
  Bus Creator/1 -> EgoLaneCenterLine02/1
  Data3/1 -> Bus Creator/4  "PC0"
  Data/1 -> Bus Creator/1  "PC3"
  Data1/1 -> Bus Creator/2  "PC2"
  Data2/1 -> Bus Creator/3  "PC1"
  Bus Selector4/2 -> Signal Copy1/1  "<dDisEnd>"
  Bus Selector4/1 -> Signal Copy2/1  "<dDisStart>"
  Signal Copy2/1 -> Data3/2, Data2/2, Data1/2, Data/2, Bus Creator/5  "dDisStart"
  Signal Copy1/1 -> Data2/3, Data1/3, Data/3, Data3/3, Bus Creator/6  "dDisEnd"
  Gain2/1 -> Data1/1  "PC2"
  Gain1/1 -> Data/1  "PC3"
  Gain3/1 -> Data2/1  "PC1"
  Gain4/1 -> Data3/1  "PC0"

== system PubIfDecisionTOS_MDL/TOS_20201112/TOS_2012080320/PP1128/AAT-AdditionalAttributes/PP_CenterLine_Calculat/EgoLane_CenterLine/EgoLaneCenterLine03 ==
  EgoLaneLine : Inport
  Add{,1..3} (4 alike) : Sum
  Bus Creator1 : BusCreator  Inputs=6
  Bus Selector : BusSelector  OutputSignals=TOS_LM_LR_Bus.LM_LR_Line03.pC0,TOS_LM_RL_Bus.LM_RL_Line03.pC0
  Bus Selector1 : BusSelector  OutputSignals=TOS_LM_LR_Bus.LM_LR_Line03.pC3,TOS_LM_RL_Bus.LM_RL_Line03.pC3
  Bus Selector2 : BusSelector  OutputSignals=TOS_LM_LR_Bus.LM_LR_Line03.pC2,TOS_LM_RL_Bus.LM_RL_Line03.pC2
  Bus Selector3 : BusSelector  OutputSignals=TOS_LM_LR_Bus.LM_LR_Line03.pC1,TOS_LM_RL_Bus.LM_RL_Line03.pC1
  Bus Selector4 : BusSelector  OutputSignals=TOS_LM_LR_Bus.LM_LR_Line03.dDisStart,TOS_LM_LR_Bus.LM_LR_Line03.dDisEnd
  Data{,1..3} (4 alike) : TOS_LIB/Data  SystemSampleTime=-1  VariantActivationTime=update diagram  Latency=0  AutoFrameSizeCalculation=off
  Gain{1..4} (4 alike) : Gain  Gain=0.5  ParamDataTypeStr=single  OutDataTypeStr=single
  Signal Copy1 : SignalConversion  OverrideOpt=off
  Signal Copy2 : SignalConversion  OverrideOpt=off
  EgoLaneCenterLine03 : Outport
  wires:
  Bus Selector/2 -> Add/2  "<pC0>"
  Add/1 -> Gain4/1
  Bus Selector/1 -> Add/1  "<pC0>"
  Bus Selector1/2 -> Add1/2  "<pC3>"
  Bus Selector3/2 -> Add3/2  "<pC1>"
  Add1/1 -> Gain1/1
  Bus Selector1/1 -> Add1/1  "<pC3>"
  Bus Selector2/2 -> Add2/2  "<pC2>"
  Add3/1 -> Gain3/1
  Bus Selector2/1 -> Add2/1  "<pC2>"
  EgoLaneLine/1 -> Bus Selector1/1, Bus Selector2/1, Bus Selector3/1, Bus Selector4/1, Bus Selector/1
  Bus Selector3/1 -> Add3/1  "<pC1>"
  Add2/1 -> Gain2/1
  Bus Creator1/1 -> EgoLaneCenterLine03/1
  Data3/1 -> Bus Creator1/4  "PC0"
  Data/1 -> Bus Creator1/1  "PC3"
  Data1/1 -> Bus Creator1/2  "PC2"
  Data2/1 -> Bus Creator1/3  "PC1"
  Bus Selector4/2 -> Signal Copy1/1  "<dDisEnd>"
  Bus Selector4/1 -> Signal Copy2/1  "<dDisStart>"
  Signal Copy1/1 -> Data3/3, Data2/3, Data1/3, Data/3, Bus Creator1/6  "dDisEnd"
  Signal Copy2/1 -> Data3/2, Data2/2, Data1/2, Data/2, Bus Creator1/5  "dDisStart"
  Gain1/1 -> Data/1  "PC3"
  Gain3/1 -> Data2/1  "PC1"
  Gain2/1 -> Data1/1  "PC2"
  Gain4/1 -> Data3/1  "PC0"

== system PubIfDecisionTOS_MDL/TOS_20201112/TOS_2012080320/PP1128/AAT-AdditionalAttributes/PP_CenterLine_Calculat/EgoLane_CenterLine/EgoLaneCenterLine04 ==
  EgoLaneLine : Inport
  Add{,1..3} (4 alike) : Sum
  Bus Creator1 : BusCreator  Inputs=6
  Bus Selector : BusSelector  OutputSignals=TOS_LM_LR_Bus.LM_LR_Line04.pC0,TOS_LM_RL_Bus.LM_RL_Line04.pC0
  Bus Selector1 : BusSelector  OutputSignals=TOS_LM_LR_Bus.LM_LR_Line04.pC3,TOS_LM_RL_Bus.LM_RL_Line04.pC3
  Bus Selector2 : BusSelector  OutputSignals=TOS_LM_LR_Bus.LM_LR_Line04.pC2,TOS_LM_RL_Bus.LM_RL_Line04.pC2
  Bus Selector3 : BusSelector  OutputSignals=TOS_LM_LR_Bus.LM_LR_Line04.pC1,TOS_LM_RL_Bus.LM_RL_Line04.pC1
  Bus Selector4 : BusSelector  OutputSignals=TOS_LM_LR_Bus.LM_LR_Line04.dDisStart,TOS_LM_LR_Bus.LM_LR_Line04.dDisEnd
  Data{,1..3} (4 alike) : TOS_LIB/Data  SystemSampleTime=-1  VariantActivationTime=update diagram  Latency=0  AutoFrameSizeCalculation=off
  Gain{1..4} (4 alike) : Gain  Gain=0.5  ParamDataTypeStr=single  OutDataTypeStr=single
  Signal Copy1 : SignalConversion  OverrideOpt=off
  Signal Copy2 : SignalConversion  OverrideOpt=off
  EgoLaneCenterLine04 : Outport
  wires:
  Bus Selector/1 -> Add/1  "<pC0>"
  Add/1 -> Gain4/1
  Bus Selector/2 -> Add/2  "<pC0>"
  Bus Selector1/2 -> Add1/2  "<pC3>"
  Bus Selector3/2 -> Add3/2  "<pC1>"
  Add1/1 -> Gain1/1
  Bus Selector1/1 -> Add1/1  "<pC3>"
  Bus Selector2/2 -> Add2/2  "<pC2>"
  Add3/1 -> Gain3/1
  Bus Selector2/1 -> Add2/1  "<pC2>"
  EgoLaneLine/1 -> Bus Selector1/1, Bus Selector2/1, Bus Selector3/1, Bus Selector4/1, Bus Selector/1
  Bus Selector3/1 -> Add3/1  "<pC1>"
  Add2/1 -> Gain2/1
  Data3/1 -> Bus Creator1/4  "PC0"
  Data/1 -> Bus Creator1/1  "PC3"
  Data1/1 -> Bus Creator1/2  "PC2"
  Data2/1 -> Bus Creator1/3  "PC1"
  Bus Creator1/1 -> EgoLaneCenterLine04/1
  Bus Selector4/2 -> Signal Copy1/1  "<dDisEnd>"
  Bus Selector4/1 -> Signal Copy2/1  "<dDisStart>"
  Gain1/1 -> Data/1  "PC3"
  Gain2/1 -> Data1/1  "PC2"
  Gain3/1 -> Data2/1  "PC1"
  Gain4/1 -> Data3/1  "PC0"
  Signal Copy2/1 -> Data3/2, Data/2, Data1/2, Data2/2, Bus Creator1/5  "dDisStart"
  Signal Copy1/1 -> Data2/3, Data1/3, Data/3, Data3/3, Bus Creator1/6  "dDisEnd"

== system PubIfDecisionTOS_MDL/TOS_20201112/TOS_2012080320/PP1128/AAT-AdditionalAttributes/PP_CenterLine_Calculat/EgoLane_CenterLine/EgoLaneCenterLine05 ==
  EgoLaneLine : Inport
  Add{,1..3} (4 alike) : Sum
  Bus Creator1 : BusCreator  Inputs=6
  Bus Selector : BusSelector  OutputSignals=TOS_LM_LR_Bus.LM_LR_Line05.pC0,TOS_LM_RL_Bus.LM_RL_Line05.pC0
  Bus Selector1 : BusSelector  OutputSignals=TOS_LM_LR_Bus.LM_LR_Line05.pC3,TOS_LM_RL_Bus.LM_RL_Line05.pC3
  Bus Selector2 : BusSelector  OutputSignals=TOS_LM_LR_Bus.LM_LR_Line05.pC2,TOS_LM_RL_Bus.LM_RL_Line05.pC2
  Bus Selector3 : BusSelector  OutputSignals=TOS_LM_LR_Bus.LM_LR_Line05.pC1,TOS_LM_RL_Bus.LM_RL_Line05.pC1
  Bus Selector4 : BusSelector  OutputSignals=TOS_LM_LR_Bus.LM_LR_Line05.dDisStart,TOS_LM_LR_Bus.LM_LR_Line05.dDisEnd
  Data{,1..3} (4 alike) : TOS_LIB/Data  SystemSampleTime=-1  VariantActivationTime=update diagram  Latency=0  AutoFrameSizeCalculation=off
  Gain{1..4} (4 alike) : Gain  Gain=0.5  ParamDataTypeStr=single  OutDataTypeStr=single
  Signal Copy1 : SignalConversion  OverrideOpt=off
  Signal Copy2 : SignalConversion  OverrideOpt=off
  EgoLaneCenterLine05 : Outport
  wires:
  Bus Selector/1 -> Add/1  "<pC0>"
  Add/1 -> Gain4/1
  Bus Selector/2 -> Add/2  "<pC0>"
  Bus Selector1/2 -> Add1/2  "<pC3>"
  Add1/1 -> Gain1/1
  Bus Selector1/1 -> Add1/1  "<pC3>"
  Bus Selector2/2 -> Add2/2  "<pC2>"
  Add3/1 -> Gain3/1
  Bus Selector2/1 -> Add2/1  "<pC2>"
  Bus Selector3/1 -> Add3/1  "<pC1>"
  Add2/1 -> Gain2/1
  Bus Selector3/2 -> Add3/2  "<pC1>"
  Data3/1 -> Bus Creator1/4  "PC0"
  Data/1 -> Bus Creator1/1  "PC3"
  Data1/1 -> Bus Creator1/2  "PC2"
  Data2/1 -> Bus Creator1/3  "PC1"
  Bus Creator1/1 -> EgoLaneCenterLine05/1
  Bus Selector4/1 -> Signal Copy2/1  "<dDisStart>"
  EgoLaneLine/1 -> Bus Selector1/1, Bus Selector2/1, Bus Selector3/1, Bus Selector4/1, Bus Selector/1
  Bus Selector4/2 -> Signal Copy1/1  "<dDisEnd>"
  Gain1/1 -> Data/1  "PC3"
  Gain3/1 -> Data2/1  "PC1"
  Gain2/1 -> Data1/1  "PC2"
  Gain4/1 -> Data3/1  "PC0"
  Signal Copy2/1 -> Data3/2, Data1/2, Data/2, Data2/2, Bus Creator1/5  "dDisStart"
  Signal Copy1/1 -> Data3/3, Data2/3, Data1/3, Data/3, Bus Creator1/6  "dDisEnd"

== system PubIfDecisionTOS_MDL/TOS_20201112/TOS_2012080320/PP1128/AAT-AdditionalAttributes/PP_CenterLine_Calculat/EgoLane_CenterLine/EgoLaneCenterLine06 ==
  EgoLaneLine : Inport
  Add{,1..3} (4 alike) : Sum
  Bus Creator1 : BusCreator  Inputs=6
  Bus Selector : BusSelector  OutputSignals=TOS_LM_LR_Bus.LM_LR_Line06.pC0,TOS_LM_RL_Bus.LM_RL_Line06.pC0
  Bus Selector1 : BusSelector  OutputSignals=TOS_LM_LR_Bus.LM_LR_Line06.pC3,TOS_LM_RL_Bus.LM_RL_Line06.pC3
  Bus Selector2 : BusSelector  OutputSignals=TOS_LM_LR_Bus.LM_LR_Line06.pC2,TOS_LM_RL_Bus.LM_RL_Line06.pC2
  Bus Selector3 : BusSelector  OutputSignals=TOS_LM_LR_Bus.LM_LR_Line06.pC1,TOS_LM_RL_Bus.LM_RL_Line06.pC1
  Bus Selector4 : BusSelector  OutputSignals=TOS_LM_LR_Bus.LM_LR_Line06.dDisStart,TOS_LM_LR_Bus.LM_LR_Line06.dDisEnd
  Data{,1..3} (4 alike) : TOS_LIB/Data  SystemSampleTime=-1  VariantActivationTime=update diagram  Latency=0  AutoFrameSizeCalculation=off
  Gain{5..8} (4 alike) : Gain  Gain=0.5  ParamDataTypeStr=single  OutDataTypeStr=single
  Signal Copy1 : SignalConversion  OverrideOpt=off
  Signal Copy2 : SignalConversion  OverrideOpt=off
  EgoLaneCenterLine06 : Outport
  wires:
  Bus Selector/1 -> Add/1  "<pC0>"
  Add/1 -> Gain8/1
  Bus Selector/2 -> Add/2  "<pC0>"
  Bus Selector1/2 -> Add1/2  "<pC3>"
  Bus Selector3/2 -> Add3/2  "<pC1>"
  Add1/1 -> Gain5/1
  Bus Selector1/1 -> Add1/1  "<pC3>"
  Bus Selector2/2 -> Add2/2  "<pC2>"
  Add3/1 -> Gain7/1
  Bus Selector2/1 -> Add2/1  "<pC2>"
  Bus Selector3/1 -> Add3/1  "<pC1>"
  Add2/1 -> Gain6/1
  Data3/1 -> Bus Creator1/4  "PC0"
  Data1/1 -> Bus Creator1/2  "PC2"
  Data2/1 -> Bus Creator1/3  "PC1"
  Bus Creator1/1 -> EgoLaneCenterLine06/1
  EgoLaneLine/1 -> Bus Selector1/1, Bus Selector2/1, Bus Selector3/1, Bus Selector4/1, Bus Selector/1
  Bus Selector4/1 -> Signal Copy2/1  "<dDisStart>"
  Bus Selector4/2 -> Signal Copy1/1  "<dDisEnd>"
  Gain5/1 -> Data/1  "PC3"
  Gain6/1 -> Data1/1  "PC2"
  Gain8/1 -> Data3/1  "PC0"
  Gain7/1 -> Data2/1  "PC1"
  Signal Copy1/1 -> Data3/3, Data2/3, Data1/3, Data/3, Bus Creator1/6  "dDisEnd"
  Signal Copy2/1 -> Data3/2, Data1/2, Data/2, Data2/2, Bus Creator1/5  "dDisStart"
  Data/1 -> Bus Creator1/1  "PC3"
